simulink model "respiratory_simulink"  (R2020a)
settings: Solver=VariableStepAuto  StartTime=0.0  StopTime=10.0  RelTol=1e-3
libraries: simulink x4
settings Model: Creator=PrasunOrchi  LastModifiedBy=PrasunOrchi

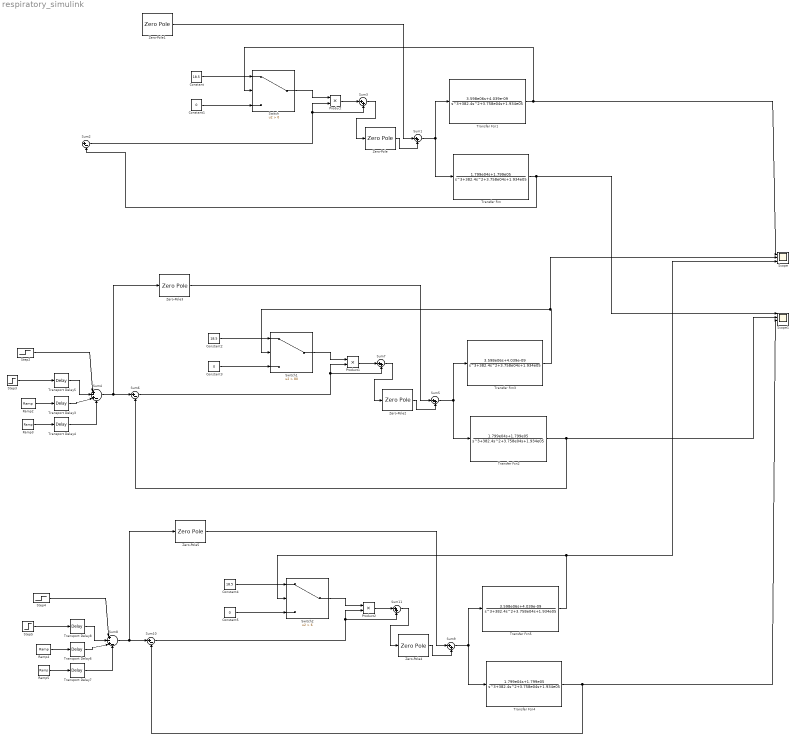
== system respiratory_simulink ==
  Constant : Constant  Value=18.5
  Constant1 : Constant  Value=0
  Constant2 : Constant  Value=18.5
  Constant3 : Constant  Value=0
  Constant4 : Constant  Value=18.5
  Constant5 : Constant  Value=0
  Product : Product
  Product1 : Product
  Product2 : Product
  Ramp{2..5} (4 alike) : simulink/Sources/Ramp  slope=750  start=0  InitialOutput=0
  Scope : Scope  NumInputPorts=3
  Scope1 : Scope  NumInputPorts=4
  Step2 : Step  Time=0.00001  After=5  SampleTime=0
  Step3 : Step  Time=0.00001  After=15  SampleTime=0
  Step4 : Step  Time=0.00001  After=5  SampleTime=0
  Step5 : Step  Time=0.00001  After=15  SampleTime=0
  Sum{1,3,5,7,9,11} (6 alike) : Sum  Inputs=|++
  Sum10 : Sum  Inputs=|+-
  Sum2 : Sum  Inputs=|+-
  Sum4 : Sum  Inputs=|+-+-
  Sum6 : Sum  Inputs=|+-
  Sum8 : Sum  Inputs=|+-+-
  Switch : Switch  Criteria=u2 > Threshold
  Switch1 : Switch  Criteria=u2 > Threshold  Threshold=80
  Switch2 : Switch  Criteria=u2 > Threshold  Threshold=6
  Transfer Fcn : TransferFcn  Numerator=[1.799e04 1.799e05]  Denominator=[1 382.4 3.758e04 1.934e05]
  Transfer Fcn1 : TransferFcn  Numerator=[3.598e06 4.039e-09]  Denominator=[1 382.4 3.758e04 1.934e05]
  Transfer Fcn2 : TransferFcn  Numerator=[1.799e04 1.799e05]  Denominator=[1 382.4 3.758e04 1.934e05]
  Transfer Fcn3 : TransferFcn  Numerator=[3.598e06 4.039e-09]  Denominator=[1 382.4 3.758e04 1.934e05]
  Transfer Fcn4 : TransferFcn  Numerator=[1.799e04 1.799e05]  Denominator=[1 382.4 3.758e04 1.934e05]
  Transfer Fcn5 : TransferFcn  Numerator=[3.598e06 4.039e-09]  Denominator=[1 382.4 3.758e04 1.934e05]
  Transport Delay3 : TransportDelay
  Transport Delay4 : TransportDelay  DelayTime=1.02
  Transport Delay5 : TransportDelay  DelayTime=5
  Transport Delay6 : TransportDelay
  Transport Delay7 : TransportDelay  DelayTime=1.02
  Transport Delay8 : TransportDelay  DelayTime=5
  Zero-Pole : ZeroPole  Zeros=[]  Poles=[0]  Gain=[0.4]
  Zero-Pole1 : ZeroPole  Zeros=[]  Poles=[]
  Zero-Pole2 : ZeroPole  Zeros=[]  Poles=[0]  Gain=[0.4]
  Zero-Pole3 : ZeroPole  Zeros=[]  Poles=[]
  Zero-Pole4 : ZeroPole  Zeros=[]  Poles=[0]  Gain=[0.4]
  Zero-Pole5 : ZeroPole  Zeros=[]  Poles=[]
  wires:
  Constant/1 -> Switch/1
  Constant1/1 -> Switch/3
  Transfer Fcn1/1 -> Scope/1, Switch/2
  Zero-Pole/1 -> Sum1/2
  Sum1/1 -> Transfer Fcn1/1, Transfer Fcn/1
  Zero-Pole1/1 -> Sum1/1
  ? -> Zero-Pole1/1, Scope1/4, Sum2/1
  Transfer Fcn/1 -> Scope1/1, Sum2/2
  Switch/1 -> Product/1
  Sum2/1 -> Sum3/2, Product/2
  Sum3/1 -> Zero-Pole/1
  Product/1 -> Sum3/1
  Sum7/1 -> Zero-Pole2/1
  Step3/1 -> Transport Delay5/1
  Constant3/1 -> Switch1/3
  Constant2/1 -> Switch1/1
  Transport Delay3/1 -> Sum4/3
  Step2/1 -> Sum4/1
  Transport Delay4/1 -> Sum4/4
  Zero-Pole2/1 -> Sum5/2
  Ramp3/1 -> Transport Delay4/1
  Transfer Fcn3/1 -> Scope/2, Switch1/2
  Sum6/1 -> Sum7/2, Product1/2
  Sum4/1 -> Zero-Pole3/1, Sum6/1
  Transport Delay5/1 -> Sum4/2
  Sum5/1 -> Transfer Fcn3/1, Transfer Fcn2/1
  Product1/1 -> Sum7/1
  Ramp2/1 -> Transport Delay3/1
  Switch1/1 -> Product1/1
  Zero-Pole3/1 -> Sum5/1
  Transfer Fcn2/1 -> Sum6/2, Scope1/2
  Sum11/1 -> Zero-Pole4/1
  Step5/1 -> Transport Delay8/1
  Constant5/1 -> Switch2/3
  Constant4/1 -> Switch2/1
  Transport Delay6/1 -> Sum8/3
  Step4/1 -> Sum8/1
  Transport Delay7/1 -> Sum8/4
  Zero-Pole4/1 -> Sum9/2
  Ramp5/1 -> Transport Delay7/1
  Transfer Fcn5/1 -> Scope/3, Switch2/2
  Sum10/1 -> Sum11/2, Product2/2
  Sum8/1 -> Zero-Pole5/1, Sum10/1
  Transport Delay8/1 -> Sum8/2
  Sum9/1 -> Transfer Fcn5/1, Transfer Fcn4/1
  Product2/1 -> Sum11/1
  Ramp4/1 -> Transport Delay6/1
  Switch2/1 -> Product2/1
  Zero-Pole5/1 -> Sum9/1
  Transfer Fcn4/1 -> Sum10/2, Scope1/3
